simulink model "H8_6GDL_partelinealizada"  (R2022b)
settings: Solver=VariableStepAuto  StartTime=0.0  StopTime=3  RelTol=1e-3
InitFcn:
  | m = 200;
  | g = 9.81;
  | 
  | x_lev12 = 0.443;
  | x_lev34 = 0.542;
  | x_guid12 = 0.4475;
  | x_guid34 = 0.5465;
  | x_lim = 0.0495;
  | 
  | y_lev13 = 0.23686;
  | y_lev24 = 0.23686;
  | y_guid13 = 0.24263;
  | y_guid24 = 0.24263;
  | y_lim = 0.0005;
  | y_brk = 0.21552;
  | 
  | z_lev = 0.08546;
  | z_guid = 0.026;
  | z_lim = 0.1055;
  | z_brk = 0.03941;
  | 
  | kp_lev = 50;
  | ki_lev = 400;
  | kp_guid = 6;
  | ki_guid = 46.5;
  | 
  | Imax_lev = 50;
  | Imin_lev = -50;
  | Imax_guid = 50;
  | Imin_guid = 0;
  | 
  | cg_nom = 0.567;
  | 
  | I = [43.082 0 0; 0 26.887 0; 0 0 29.297]
undefined symbols (not defined in the file or in its folder): ems, hems
libraries: shared6dof x1
settings Model: Creator=aceao  LastModifiedBy=aceao

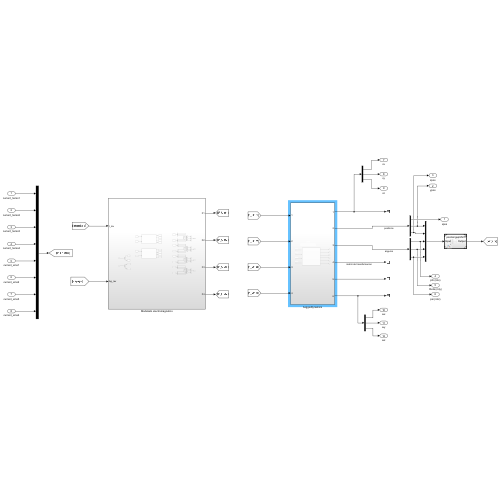
[thumbnail: Simulink's stored preview of the top-level diagram]
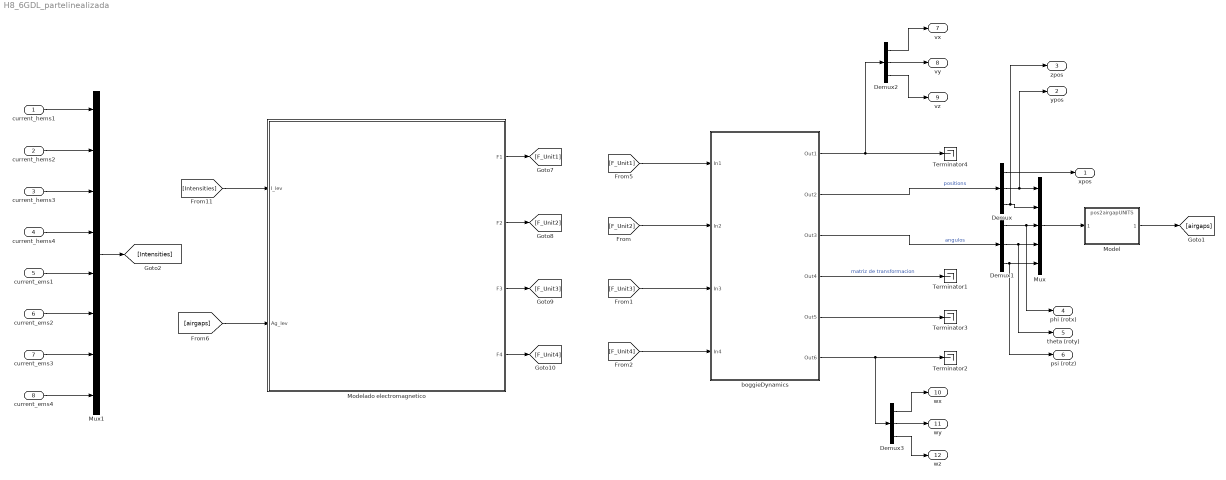
== system H8_6GDL_partelinealizada ==
  current_hems1 : Inport
  current_hems2 : Inport  Port=2
  current_hems3 : Inport  Port=3
  current_hems4 : Inport  Port=4
  current_ems1 : Inport  Port=5
  current_ems2 : Inport  Port=6
  current_ems3 : Inport  Port=7
  current_ems4 : Inport  Port=8
  Demux{,1..3} (4 alike) : Demux  Outputs=3
  Model : ModelReference  ModelNameDialog=pos2airgapUNITS.slx  SimulationMode=Normal  ModelReferenceVersion=1.2
  Modelado electromagnetico : Subsystem
  Mux : Mux  Inputs=5
  Mux1 : Mux  Inputs=8
  Terminator{1..4} (4 alike) : Terminator
  boggieDynamics : Subsystem
  xpos : Outport
  ypos : Outport  Port=2
  zpos : Outport  Port=3
  phi (rotx) : Outport  Port=4
  theta (roty) : Outport  Port=5
  psi (rotz) : Outport  Port=6
  vx : Outport  Port=7
  vy : Outport  Port=8
  vz : Outport  Port=9
  wx : Outport  Port=10
  wy : Outport  Port=11
  wz : Outport  Port=12
  wires:
  Mux1/1 -> [Intensities]
  current_hems2/1 -> Mux1/2
  current_ems3/1 -> Mux1/7
  current_hems4/1 -> Mux1/4
  Modelado electromagnetico/4(F4) -> [F_Unit4]
  current_ems2/1 -> Mux1/6
  current_hems3/1 -> Mux1/3
  current_ems1/1 -> Mux1/5
  current_ems4/1 -> Mux1/8
  current_hems1/1 -> Mux1/1
  Modelado electromagnetico/2(F2) -> [F_Unit2]
  [Intensities] -> Modelado electromagnetico/1(I_lev)
  Modelado electromagnetico/1(F1) -> [F_Unit1]
  Modelado electromagnetico/3(F3) -> [F_Unit3]
  [airgaps] -> Modelado electromagnetico/2(Ag_lev)
  boggieDynamics/2(Out2) -> Demux/1  "positions"
  boggieDynamics/5(Out5) -> Terminator3/1
  Demux1/3 -> psi (rotz)/1, Mux/5
  boggieDynamics/3(Out3) -> Demux1/1  "angulos"
  boggieDynamics/6(Out6) -> Terminator2/1, Demux3/1
  Demux/3 -> zpos/1, Mux/2
  [F_Unit1] -> boggieDynamics/1(In1)
  [F_Unit3] -> boggieDynamics/3(In3)
  Demux/1 -> xpos/1
  boggieDynamics/1(Out1) -> Terminator4/1, Demux2/1
  Mux/1 -> Model/1
  Demux/2 -> Mux/1, ypos/1
  Demux1/1 -> phi (rotx)/1, Mux/3
  [F_Unit2] -> boggieDynamics/2(In2)
  Demux1/2 -> theta (roty)/1, Mux/4
  [F_Unit4] -> boggieDynamics/4(In4)
  boggieDynamics/4(Out4) -> Terminator1/1  "matriz de transformacion"
  Demux2/2 -> vy/1
  Demux2/3 -> vz/1
  Demux3/1 -> wx/1
  Demux3/2 -> wy/1
  Demux3/3 -> wz/1
  Demux2/1 -> vx/1
  Model/1 -> [airgaps]

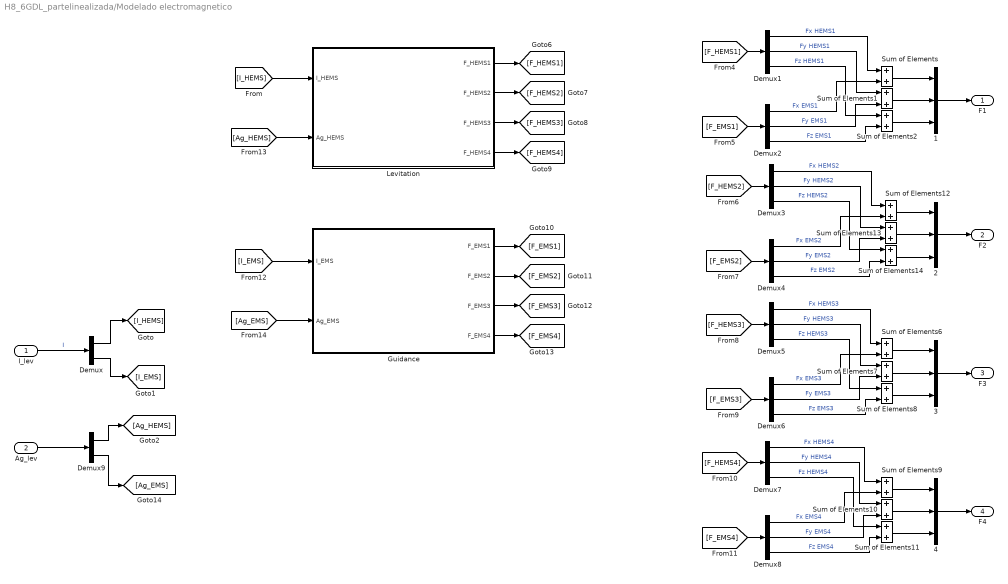
== system H8_6GDL_partelinealizada/Modelado electromagnetico ==
  I_lev : Inport
  Ag_lev : Inport  Port=2
  {1..4} (4 alike) : Mux  Inputs=3
  Demux : Demux  Outputs=2
  Demux{1..8} (8 alike) : Demux  Outputs=3
  Demux9 : Demux  Outputs=2
  Guidance : Subsystem
  Levitation : Subsystem
  Sum of Elements{,1..2,6..14} (12 alike) : Sum
  F1 : Outport
  F2 : Outport  Port=2
  F3 : Outport  Port=3
  F4 : Outport  Port=4
  wires:
  I_lev/1 -> Demux/1  "I"
  Demux/1 -> [I_HEMS]
  Demux/2 -> [I_EMS]
  [I_HEMS] -> Levitation/1(I_HEMS)
  Levitation/1(F_HEMS1) -> [F_HEMS1]
  Levitation/2(F_HEMS2) -> [F_HEMS2]
  Levitation/3(F_HEMS3) -> [F_HEMS3]
  Levitation/4(F_HEMS4) -> [F_HEMS4]
  Sum of Elements/1 -> 1/1
  1/1 -> F1/1
  Sum of Elements1/1 -> 1/2
  Sum of Elements2/1 -> 1/3
  2/1 -> F2/1
  [F_HEMS1] -> Demux1/1
  Demux1/1 -> Sum of Elements/1  "Fx HEMS1"
  Demux1/2 -> Sum of Elements1/1  "Fy HEMS1"
  Demux1/3 -> Sum of Elements2/1  "Fz HEMS1"
  3/1 -> F3/1
  Sum of Elements8/1 -> 3/3
  Sum of Elements6/1 -> 3/1
  Sum of Elements7/1 -> 3/2
  4/1 -> F4/1
  Sum of Elements11/1 -> 4/3
  Sum of Elements9/1 -> 4/1
  Sum of Elements10/1 -> 4/2
  Guidance/2(F_EMS2) -> [F_EMS2]
  Guidance/3(F_EMS3) -> [F_EMS3]
  Guidance/4(F_EMS4) -> [F_EMS4]
  Guidance/1(F_EMS1) -> [F_EMS1]
  Demux2/1 -> Sum of Elements/2  "Fx EMS1"
  [F_EMS1] -> Demux2/1
  Demux2/2 -> Sum of Elements1/2  "Fy EMS1"
  Demux2/3 -> Sum of Elements2/2  "Fz EMS1"
  [F_EMS2] -> Demux4/1
  Demux4/1 -> Sum of Elements12/2  "Fx EMS2"
  Demux4/2 -> Sum of Elements13/2  "Fy EMS2"
  Sum of Elements14/1 -> 2/3
  Demux3/1 -> Sum of Elements12/1  "Fx HEMS2"
  [F_HEMS2] -> Demux3/1
  Demux3/2 -> Sum of Elements13/1  "Fy HEMS2"
  Demux3/3 -> Sum of Elements14/1  "Fz HEMS2"
  Sum of Elements13/1 -> 2/2
  Sum of Elements12/1 -> 2/1
  Demux4/3 -> Sum of Elements14/2  "Fz EMS2"
  Demux5/3 -> Sum of Elements8/1  "Fz HEMS3"
  Demux5/2 -> Sum of Elements7/1  "Fy HEMS3"
  [F_HEMS3] -> Demux5/1
  Demux6/3 -> Sum of Elements8/2  "Fz EMS3"
  [F_EMS3] -> Demux6/1
  Demux6/1 -> Sum of Elements6/2  "Fx EMS3"
  Demux5/1 -> Sum of Elements6/1  "Fx HEMS3"
  Demux6/2 -> Sum of Elements7/2  "Fy EMS3"
  Demux7/3 -> Sum of Elements11/1  "Fz HEMS4"
  Demux8/3 -> Sum of Elements11/2  "Fz EMS4"
  Demux8/2 -> Sum of Elements10/2  "Fy EMS4"
  Demux7/2 -> Sum of Elements10/1  "Fy HEMS4"
  Demux7/1 -> Sum of Elements9/1  "Fx HEMS4"
  Demux8/1 -> Sum of Elements9/2  "Fx EMS4"
  [F_HEMS4] -> Demux7/1
  [F_EMS4] -> Demux8/1
  [I_EMS] -> Guidance/1(I_EMS)
  Ag_lev/1 -> Demux9/1
  Demux9/1 -> [Ag_HEMS]
  Demux9/2 -> [Ag_EMS]
  [Ag_HEMS] -> Levitation/2(Ag_HEMS)
  [Ag_EMS] -> Guidance/2(Ag_EMS)

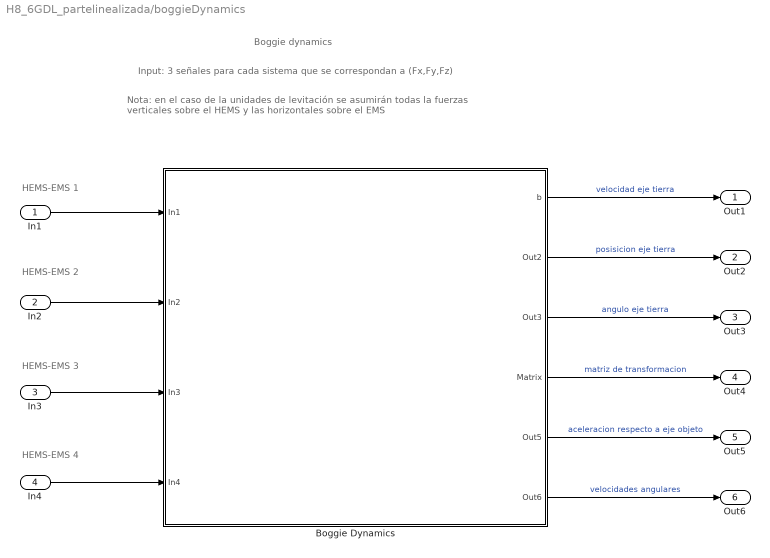
== system H8_6GDL_partelinealizada/boggieDynamics ==
  note: Input: 3 señales para cada sistema que se correspondan a (Fx,Fy,Fz)
  note: HEMS-EMS 3
  note: HEMS-EMS 1
  note: HEMS-EMS 4
  note: HEMS-EMS 2
  note: Boggie dynamics
  note: Nota: en el caso de la unidades de levitación se asumirán todas la fuerzas
      | verticales sobre el HEMS y las horizontales sobre el EMS
  In1 : Inport
  In2 : Inport  Port=2
  In3 : Inport  Port=3
  In4 : Inport  Port=4
  Boggie Dynamics : Subsystem
      mask Display: image('C:\UPV\Hyperloop\Levitacion\ejes.png'); % Use "Edit Image" on toolstrip to change.
  Out1 : Outport
  Out2 : Outport  Port=2
  Out3 : Outport  Port=3
  Out4 : Outport  Port=4
  Out5 : Outport  Port=5
  Out6 : Outport  Port=6
  wires:
  Boggie Dynamics/4(Matrix) -> Out4/1  "matriz de transformacion"
  Boggie Dynamics/6(Out6) -> Out6/1  "velocidades angulares"
  Boggie Dynamics/5(Out5) -> Out5/1  "aceleracion respecto a eje objeto"
  In1/1 -> Boggie Dynamics/1(In1)
  In3/1 -> Boggie Dynamics/3(In3)
  In4/1 -> Boggie Dynamics/4(In4)
  Boggie Dynamics/1(b) -> Out1/1  "velocidad eje tierra"
  In2/1 -> Boggie Dynamics/2(In2)
  Boggie Dynamics/2(Out2) -> Out2/1  "posisicion eje tierra"
  Boggie Dynamics/3(Out3) -> Out3/1  "angulo eje tierra"

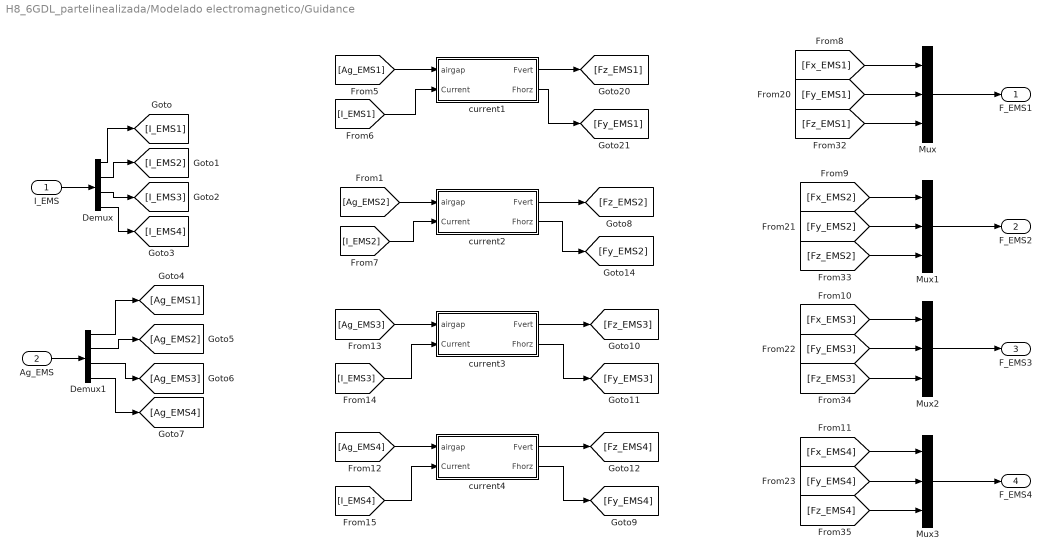
== system H8_6GDL_partelinealizada/Modelado electromagnetico/Guidance ==
  I_EMS : Inport
  Ag_EMS : Inport  Port=2
  Demux : Demux
  Demux1 : Demux
  Mux{,1..3} (4 alike) : Mux  Inputs=3
  current1 : Subsystem
  current2 : Subsystem
  current3 : Subsystem
  current4 : Subsystem
  F_EMS1 : Outport
  F_EMS2 : Outport  Port=2
  F_EMS3 : Outport  Port=3
  F_EMS4 : Outport  Port=4
  wires:
  [Fz_EMS4] -> Mux3/3
  Demux1/4 -> [Ag_EMS4]
  [Fy_EMS1] -> Mux/2
  I_EMS/1 -> Demux/1
  Mux1/1 -> F_EMS2/1
  Demux/2 -> [I_EMS2]
  [Fy_EMS3] -> Mux2/2
  Mux3/1 -> F_EMS4/1
  [Fy_EMS4] -> Mux3/2
  [Fz_EMS1] -> Mux/3
  Mux/1 -> F_EMS1/1
  Mux2/1 -> F_EMS3/1
  [Fx_EMS3] -> Mux2/1
  Demux1/3 -> [Ag_EMS3]
  Ag_EMS/1 -> Demux1/1
  [Fz_EMS3] -> Mux2/3
  Demux/1 -> [I_EMS1]
  [Fz_EMS2] -> Mux1/3
  [Fx_EMS1] -> Mux/1
  Demux1/1 -> [Ag_EMS1]
  Demux/4 -> [I_EMS4]
  [Fx_EMS2] -> Mux1/1
  [Fy_EMS2] -> Mux1/2
  [Fx_EMS4] -> Mux3/1
  Demux/3 -> [I_EMS3]
  Demux1/2 -> [Ag_EMS2]
  current1/1(Fvert) -> [Fz_EMS1]
  current1/2(Fhorz) -> [Fy_EMS1]
  [Ag_EMS1] -> current1/1(airgap)
  [I_EMS1] -> current1/2(Current)
  current2/1(Fvert) -> [Fz_EMS2]
  [Ag_EMS2] -> current2/1(airgap)
  [I_EMS2] -> current2/2(Current)
  current2/2(Fhorz) -> [Fy_EMS2]
  current3/1(Fvert) -> [Fz_EMS3]
  [Ag_EMS3] -> current3/1(airgap)
  current4/1(Fvert) -> [Fz_EMS4]
  [I_EMS3] -> current3/2(Current)
  current4/2(Fhorz) -> [Fy_EMS4]
  current3/2(Fhorz) -> [Fy_EMS3]
  [Ag_EMS4] -> current4/1(airgap)
  [I_EMS4] -> current4/2(Current)

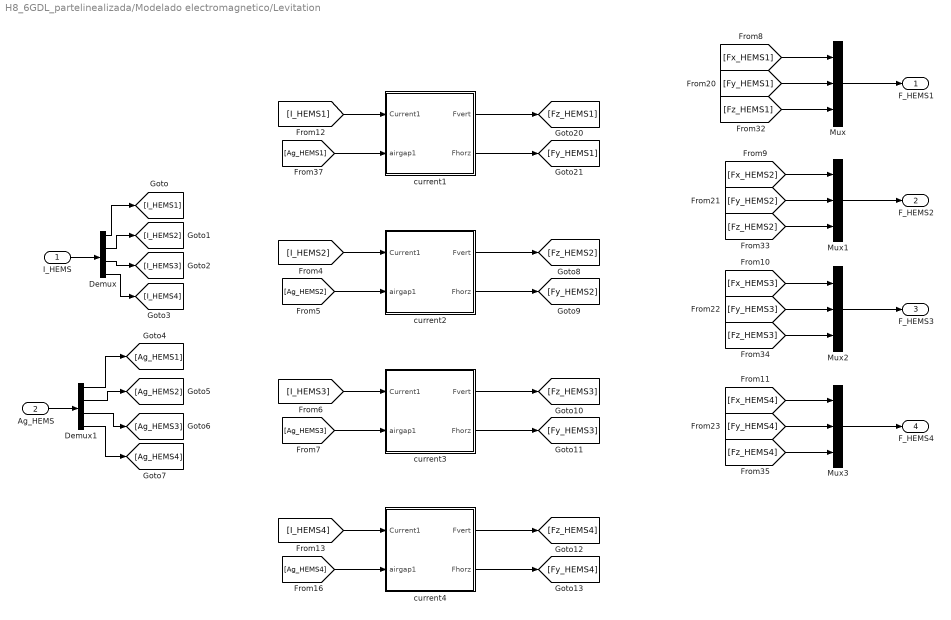
== system H8_6GDL_partelinealizada/Modelado electromagnetico/Levitation ==
  I_HEMS : Inport
  Ag_HEMS : Inport  Port=2
  Demux : Demux
  Demux1 : Demux
  Mux{,1..3} (4 alike) : Mux  Inputs=3
  current1 : Subsystem
  current2 : Subsystem
  current3 : Subsystem
  current4 : Subsystem
  F_HEMS1 : Outport
  F_HEMS2 : Outport  Port=2
  F_HEMS3 : Outport  Port=3
  F_HEMS4 : Outport  Port=4
  wires:
  I_HEMS/1 -> Demux/1
  Mux/1 -> F_HEMS1/1
  Mux1/1 -> F_HEMS2/1
  Mux2/1 -> F_HEMS3/1
  Mux3/1 -> F_HEMS4/1
  Demux/1 -> [I_HEMS1]
  Demux/2 -> [I_HEMS2]
  Demux/3 -> [I_HEMS3]
  Demux/4 -> [I_HEMS4]
  Demux1/2 -> [Ag_HEMS2]
  Demux1/3 -> [Ag_HEMS3]
  Ag_HEMS/1 -> Demux1/1
  Demux1/4 -> [Ag_HEMS4]
  Demux1/1 -> [Ag_HEMS1]
  [Fx_HEMS1] -> Mux/1
  [Fx_HEMS2] -> Mux1/1
  [Fx_HEMS3] -> Mux2/1
  [Fx_HEMS4] -> Mux3/1
  [Fy_HEMS1] -> Mux/2
  [Fy_HEMS2] -> Mux1/2
  [Fy_HEMS3] -> Mux2/2
  [Fy_HEMS4] -> Mux3/2
  [Fz_HEMS1] -> Mux/3
  [Fz_HEMS2] -> Mux1/3
  [Fz_HEMS3] -> Mux2/3
  [Fz_HEMS4] -> Mux3/3
  current1/1(Fvert) -> [Fz_HEMS1]
  current1/2(Fhorz) -> [Fy_HEMS1]
  [I_HEMS1] -> current1/1(Current1)
  [Ag_HEMS1] -> current1/2(airgap1)
  current2/1(Fvert) -> [Fz_HEMS2]
  [Ag_HEMS2] -> current2/2(airgap1)
  current2/2(Fhorz) -> [Fy_HEMS2]
  [I_HEMS2] -> current2/1(Current1)
  current3/1(Fvert) -> [Fz_HEMS3]
  [Ag_HEMS3] -> current3/2(airgap1)
  [I_HEMS4] -> current4/1(Current1)
  [I_HEMS3] -> current3/1(Current1)
  current4/2(Fhorz) -> [Fy_HEMS4]
  current3/2(Fhorz) -> [Fy_HEMS3]
  current4/1(Fvert) -> [Fz_HEMS4]
  [Ag_HEMS4] -> current4/2(airgap1)

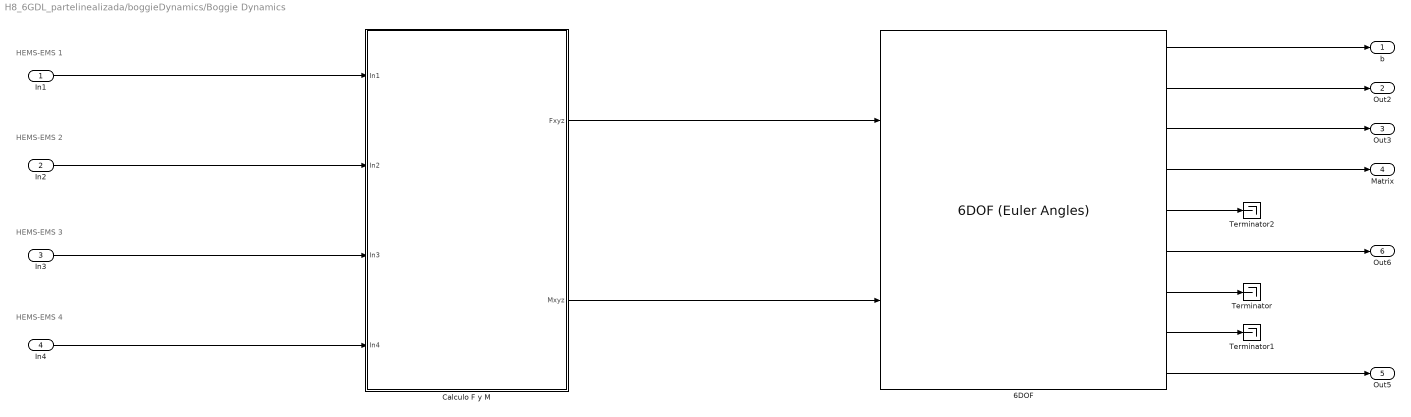
== system H8_6GDL_partelinealizada/boggieDynamics/Boggie Dynamics ==
  note: HEMS-EMS 1
  note: HEMS-EMS 2
  note: HEMS-EMS 3
  note: HEMS-EMS 4
  In1 : Inport
  In2 : Inport  Port=2
  In3 : Inport  Port=3
  In4 : Inport  Port=4
  "6DOF " : shared6dof/6DOF (Euler Angles)  units=Metric (MKS)  mtype=Fixed  rep=Euler Angles  xme_0=[0 0 cg_nom]  Vm_0=[0 0 0]  eul_0=[0 0 0]  pm_0=[0 0 0]  mass_0=m  mass_e=0.5  mass_f=2.0  inertia=I  inertia_e=eye(3)  inertia_f=2*eye(3)  k_quat=1.0  vre_flag=on  abi_flag=on  aMode=0  xme_statename=''  Vm_statename=''  eul_statename=''  quat_statename=''  pm_statename=''  mass_statename=''
  Calculo F y M : Subsystem
  Terminator : Terminator
  Terminator1 : Terminator
  Terminator2 : Terminator
  b : Outport
  Out2 : Outport  Port=2
  Out3 : Outport  Port=3
  Matrix : Outport  Port=4
  Out5 : Outport  Port=5
  Out6 : Outport  Port=6
  wires:
  "6DOF "/1 -> b/1
  "6DOF "/2 -> Out2/1
  "6DOF "/3 -> Out3/1
  In1/1 -> Calculo F y M/1(In1)
  In2/1 -> Calculo F y M/2(In2)
  In3/1 -> Calculo F y M/3(In3)
  In4/1 -> Calculo F y M/4(In4)
  "6DOF "/6 -> Out6/1
  "6DOF "/8 -> Terminator1/1
  "6DOF "/7 -> Terminator/1
  Calculo F y M/1(Fxyz) -> "6DOF "/1
  Calculo F y M/2(Mxyz) -> "6DOF "/2
  "6DOF "/4 -> Matrix/1
  "6DOF "/9 -> Out5/1
  "6DOF "/5 -> Terminator2/1

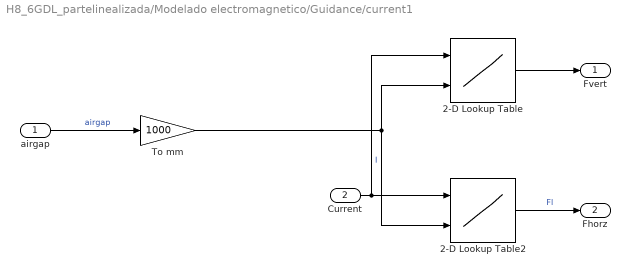
== system H8_6GDL_partelinealizada/Modelado electromagnetico/Guidance/current1 ==
  airgap : Inport
  Current : Inport  Port=2
  2-D Lookup Table : Lookup_n-D  BreakpointsForDimension1=ems.Current  BreakpointsForDimension2=ems.Airgap'  Table=ems.Force_Vertical  InternalRulePriority=Speed  RndMeth=Simplest
      settings: InputPortMap=u0,u1
  2-D Lookup Table2 : Lookup_n-D  BreakpointsForDimension1=ems.Current  BreakpointsForDimension2=ems.Airgap'  Table=ems.Force_Horizontal  InternalRulePriority=Speed  RndMeth=Simplest
      settings: InputPortMap=u0,u1
  To mm : Gain  Gain=1000
  Fvert : Outport
  Fhorz : Outport  Port=2
  wires:
  2-D Lookup Table2/1 -> Fhorz/1  "Fl"
  Current/1 -> 2-D Lookup Table2/1, 2-D Lookup Table/1  "I"
  2-D Lookup Table/1 -> Fvert/1
  airgap/1 -> To mm/1  "airgap"
  To mm/1 -> 2-D Lookup Table/2, 2-D Lookup Table2/2

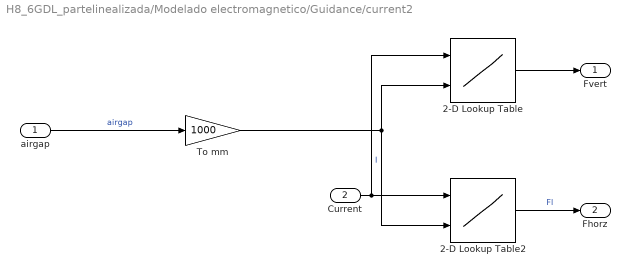
== system H8_6GDL_partelinealizada/Modelado electromagnetico/Guidance/current2 ==
  airgap : Inport
  Current : Inport  Port=2
  2-D Lookup Table : Lookup_n-D  BreakpointsForDimension1=ems.Current  BreakpointsForDimension2=ems.Airgap'  Table=ems.Force_Vertical  InternalRulePriority=Speed  RndMeth=Simplest
      settings: InputPortMap=u0,u1
  2-D Lookup Table2 : Lookup_n-D  BreakpointsForDimension1=ems.Current  BreakpointsForDimension2=ems.Airgap'  Table=ems.Force_Horizontal  InternalRulePriority=Speed  RndMeth=Simplest
      settings: InputPortMap=u0,u1
  To mm : Gain  Gain=1000
  Fvert : Outport
  Fhorz : Outport  Port=2
  wires:
  2-D Lookup Table2/1 -> Fhorz/1  "Fl"
  Current/1 -> 2-D Lookup Table2/1, 2-D Lookup Table/1  "I"
  2-D Lookup Table/1 -> Fvert/1
  airgap/1 -> To mm/1  "airgap"
  To mm/1 -> 2-D Lookup Table2/2, 2-D Lookup Table/2

== system H8_6GDL_partelinealizada/Modelado electromagnetico/Guidance/current3 ==
  airgap : Inport
  Current : Inport  Port=2
  2-D Lookup Table : Lookup_n-D  BreakpointsForDimension1=ems.Current  BreakpointsForDimension2=ems.Airgap'  Table=ems.Force_Vertical  InternalRulePriority=Speed  RndMeth=Simplest
      settings: InputPortMap=u0,u1
  2-D Lookup Table2 : Lookup_n-D  BreakpointsForDimension1=ems.Current  BreakpointsForDimension2=ems.Airgap'  Table=ems.Force_Horizontal  InternalRulePriority=Speed  RndMeth=Simplest
      settings: InputPortMap=u0,u1
  To mm : Gain  Gain=1000
  Fvert : Outport
  Fhorz : Outport  Port=2
  wires:
  2-D Lookup Table2/1 -> Fhorz/1  "Fl"
  Current/1 -> 2-D Lookup Table2/1, 2-D Lookup Table/1  "I"
  2-D Lookup Table/1 -> Fvert/1
  airgap/1 -> To mm/1  "airgap"
  To mm/1 -> 2-D Lookup Table/2, 2-D Lookup Table2/2

== system H8_6GDL_partelinealizada/Modelado electromagnetico/Guidance/current4 ==
  airgap : Inport
  Current : Inport  Port=2
  2-D Lookup Table : Lookup_n-D  BreakpointsForDimension1=ems.Current  BreakpointsForDimension2=ems.Airgap'  Table=ems.Force_Vertical  InternalRulePriority=Speed  RndMeth=Simplest
      settings: InputPortMap=u0,u1
  2-D Lookup Table2 : Lookup_n-D  BreakpointsForDimension1=ems.Current  BreakpointsForDimension2=ems.Airgap'  Table=ems.Force_Horizontal  InternalRulePriority=Speed  RndMeth=Simplest
      settings: InputPortMap=u0,u1
  To mm : Gain  Gain=1000
  Fvert : Outport
  Fhorz : Outport  Port=2
  wires:
  2-D Lookup Table2/1 -> Fhorz/1  "Fl"
  Current/1 -> 2-D Lookup Table2/1, 2-D Lookup Table/1  "I"
  2-D Lookup Table/1 -> Fvert/1
  airgap/1 -> To mm/1  "airgap"
  To mm/1 -> 2-D Lookup Table/2, 2-D Lookup Table2/2

== system H8_6GDL_partelinealizada/Modelado electromagnetico/Levitation/current1 ==
  Current1 : Inport
  airgap1 : Inport  Port=2
  2-D Lookup Table : Lookup_n-D  BreakpointsForDimension1=hems.Airgap'  BreakpointsForDimension2=hems.Current  Table=hems.Force_Vertical  InternalRulePriority=Speed  RndMeth=Simplest
      settings: InputPortMap=u0,u1
  2-D Lookup Table1 : Lookup_n-D  BreakpointsForDimension1=hems.Airgap'  BreakpointsForDimension2=hems.Current  Table=hems.Force_Horizontal  InternalRulePriority=Speed  RndMeth=Simplest
      settings: InputPortMap=u0,u1
  To mm : Gain  Gain=1000
  Fvert : Outport
  Fhorz : Outport  Port=2
  wires:
  2-D Lookup Table1/1 -> Fhorz/1  "Fl"
  2-D Lookup Table/1 -> Fvert/1  "Fl"
  Current1/1 -> 2-D Lookup Table1/2, 2-D Lookup Table/2  "I"
  airgap1/1 -> To mm/1
  To mm/1 -> 2-D Lookup Table1/1, 2-D Lookup Table/1

== system H8_6GDL_partelinealizada/Modelado electromagnetico/Levitation/current2 ==
  Current1 : Inport
  airgap1 : Inport  Port=2
  2-D Lookup Table : Lookup_n-D  BreakpointsForDimension1=hems.Airgap'  BreakpointsForDimension2=hems.Current  Table=hems.Force_Vertical  InternalRulePriority=Speed  RndMeth=Simplest
      settings: InputPortMap=u0,u1
  2-D Lookup Table1 : Lookup_n-D  BreakpointsForDimension1=hems.Airgap'  BreakpointsForDimension2=hems.Current  Table=hems.Force_Horizontal  InternalRulePriority=Speed  RndMeth=Simplest
      settings: InputPortMap=u0,u1
  To mm : Gain  Gain=1000
  Fvert : Outport
  Fhorz : Outport  Port=2
  wires:
  2-D Lookup Table1/1 -> Fhorz/1  "Fl"
  2-D Lookup Table/1 -> Fvert/1  "Fl"
  Current1/1 -> 2-D Lookup Table1/2, 2-D Lookup Table/2  "I"
  airgap1/1 -> To mm/1
  To mm/1 -> 2-D Lookup Table1/1, 2-D Lookup Table/1

== system H8_6GDL_partelinealizada/Modelado electromagnetico/Levitation/current3 ==
  Current1 : Inport
  airgap1 : Inport  Port=2
  2-D Lookup Table : Lookup_n-D  BreakpointsForDimension1=hems.Airgap'  BreakpointsForDimension2=hems.Current  Table=hems.Force_Vertical  InternalRulePriority=Speed  RndMeth=Simplest
      settings: InputPortMap=u0,u1
  2-D Lookup Table1 : Lookup_n-D  BreakpointsForDimension1=hems.Airgap'  BreakpointsForDimension2=hems.Current  Table=hems.Force_Horizontal  InternalRulePriority=Speed  RndMeth=Simplest
      settings: InputPortMap=u0,u1
  To mm : Gain  Gain=1000
  Fvert : Outport
  Fhorz : Outport  Port=2
  wires:
  2-D Lookup Table1/1 -> Fhorz/1  "Fl"
  2-D Lookup Table/1 -> Fvert/1  "Fl"
  Current1/1 -> 2-D Lookup Table1/2, 2-D Lookup Table/2  "I"
  airgap1/1 -> To mm/1
  To mm/1 -> 2-D Lookup Table1/1, 2-D Lookup Table/1

== system H8_6GDL_partelinealizada/Modelado electromagnetico/Levitation/current4 ==
  Current1 : Inport
  airgap1 : Inport  Port=2
  2-D Lookup Table : Lookup_n-D  BreakpointsForDimension1=hems.Airgap'  BreakpointsForDimension2=hems.Current  Table=hems.Force_Vertical  InternalRulePriority=Speed  RndMeth=Simplest
      settings: InputPortMap=u0,u1
  2-D Lookup Table1 : Lookup_n-D  BreakpointsForDimension1=hems.Airgap'  BreakpointsForDimension2=hems.Current  Table=hems.Force_Horizontal  InternalRulePriority=Speed  RndMeth=Simplest
      settings: InputPortMap=u0,u1
  To mm : Gain  Gain=1000
  Fvert : Outport
  Fhorz : Outport  Port=2
  wires:
  2-D Lookup Table1/1 -> Fhorz/1  "Fl"
  2-D Lookup Table/1 -> Fvert/1  "Fl"
  Current1/1 -> 2-D Lookup Table1/2, 2-D Lookup Table/2  "I"
  airgap1/1 -> To mm/1
  To mm/1 -> 2-D Lookup Table1/1, 2-D Lookup Table/1

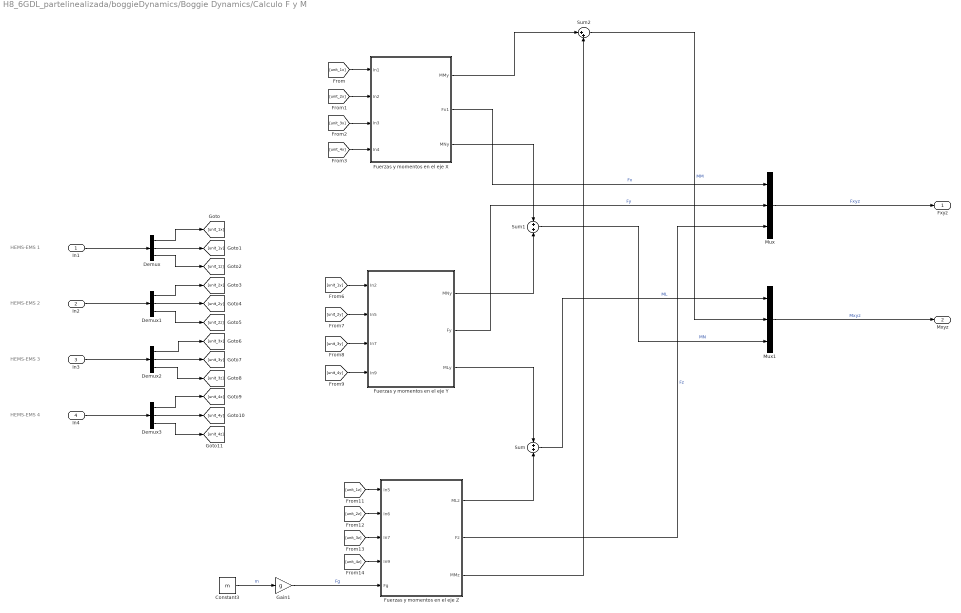
== system H8_6GDL_partelinealizada/boggieDynamics/Boggie Dynamics/Calculo F y M ==
  note: HEMS-EMS 3
  note: HEMS-EMS 1
  note: HEMS-EMS 4
  note: HEMS-EMS 2
  In1 : Inport
  In2 : Inport  Port=2
  In3 : Inport  Port=3
  In4 : Inport  Port=4
  Constant3 : Constant  Value=m
  Demux{,1..3} (4 alike) : Demux  Outputs=3
  Fuerzas y momentos en el eje X : Subsystem
  Fuerzas y momentos en el eje Y : Subsystem
  Fuerzas y momentos en el eje Z : Subsystem
  Gain1 : Gain  Gain=g
  Mux : Mux  Inputs=3
  Mux1 : Mux  Inputs=3
  Sum : Sum
  Sum1 : Sum
  Sum2 : Sum  Inputs=|++
  Fxyz : Outport
  Mxyz : Outport  Port=2
  wires:
  In3/1 -> Demux2/1
  Constant3/1 -> Gain1/1  "m"
  Sum2/1 -> Mux1/2  "MM"
  Mux/1 -> Fxyz/1  "Fxyz"
  In4/1 -> Demux3/1
  Mux1/1 -> Mxyz/1  "Mxyz"
  Sum1/1 -> Mux1/3  "MN"
  Sum/1 -> Mux1/1  "ML"
  In2/1 -> Demux1/1
  In1/1 -> Demux/1
  Fuerzas y momentos en el eje X/1(MMy) -> Sum2/1
  Fuerzas y momentos en el eje X/2(Fx1) -> Mux/1  "Fx"
  Fuerzas y momentos en el eje X/3(MNy) -> Sum1/1
  Fuerzas y momentos en el eje Y/2(Fy) -> Mux/2  "Fy"
  Fuerzas y momentos en el eje Y/1(MNy) -> Sum1/2
  Fuerzas y momentos en el eje Y/3(MLy) -> Sum/1
  Gain1/1 -> Fuerzas y momentos en el eje Z/5(Fg)  "Fg"
  Fuerzas y momentos en el eje Z/2(Fz) -> Mux/3  "Fz"
  Fuerzas y momentos en el eje Z/1(MLz) -> Sum/2
  Demux3/1 -> [unit_4x]
  Demux3/2 -> [unit_4y]
  Demux3/3 -> [unit_4z]
  Demux2/1 -> [unit_3x]
  Demux2/2 -> [unit_3y]
  Demux2/3 -> [unit_3z]
  Demux1/1 -> [unit_2x]
  Demux1/2 -> [unit_2y]
  Demux1/3 -> [unit_2z]
  Demux/1 -> [unit_1x]
  Demux/2 -> [unit_1y]
  Demux/3 -> [unit_1z]
  [unit_1x] -> Fuerzas y momentos en el eje X/1(In1)
  [unit_2x] -> Fuerzas y momentos en el eje X/2(In2)
  [unit_3x] -> Fuerzas y momentos en el eje X/3(In3)
  [unit_4x] -> Fuerzas y momentos en el eje X/4(In4)
  [unit_4y] -> Fuerzas y momentos en el eje Y/4(In9)
  [unit_1y] -> Fuerzas y momentos en el eje Y/1(In2)
  [unit_2y] -> Fuerzas y momentos en el eje Y/2(In5)
  [unit_3y] -> Fuerzas y momentos en el eje Y/3(In7)
  [unit_1z] -> Fuerzas y momentos en el eje Z/1(In5)
  [unit_3z] -> Fuerzas y momentos en el eje Z/3(In7)
  [unit_2z] -> Fuerzas y momentos en el eje Z/2(In6)
  [unit_4z] -> Fuerzas y momentos en el eje Z/4(In9)
  Fuerzas y momentos en el eje Z/3(MMz) -> Sum2/2

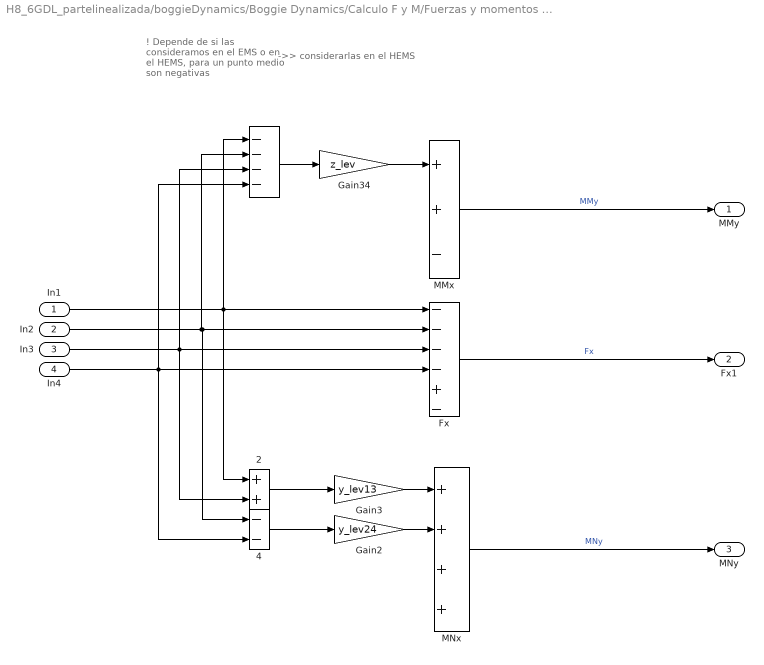
== system H8_6GDL_partelinealizada/boggieDynamics/Boggie Dynamics/Calculo F y M/Fuerzas y momentos en el eje X ==
  note: ! Depende de si las consideramos en el EMS o en el HEMS,
      | para un punto medio son negativas
  note: ->> considerarlas en el HEMS
  In1 : Inport
  In2 : Inport  Port=2
  In3 : Inport  Port=3
  In4 : Inport  Port=4
  " " : Sum  Inputs=----
  " 2" : Sum
  " 4" : Sum  Inputs=--
  Fx : Sum  Inputs=----+-
  Gain2 : Gain  Gain=y_lev24
  Gain3 : Gain  Gain=y_lev13
  Gain34 : Gain  Gain=z_lev
  MMx : Sum  Inputs=++-
  MNx : Sum  Inputs=++++
  MMy : Outport
  Fx1 : Outport  Port=2
  MNy : Outport  Port=3
  wires:
  In1/1 -> " 2"/1, " "/1, Fx/1
  In2/1 -> " "/2, " 4"/1, Fx/2
  Fx/1 -> Fx1/1  "Fx"
  MMx/1 -> MMy/1  "MMy"
  In4/1 -> " 4"/2, " "/4, Fx/4
  In3/1 -> " "/3, " 2"/2, Fx/3
  Gain34/1 -> MMx/1
  MNx/1 -> MNy/1  "MNy"
  " "/1 -> Gain34/1
  " 4"/1 -> Gain2/1
  " 2"/1 -> Gain3/1
  Gain3/1 -> MNx/1
  Gain2/1 -> MNx/2

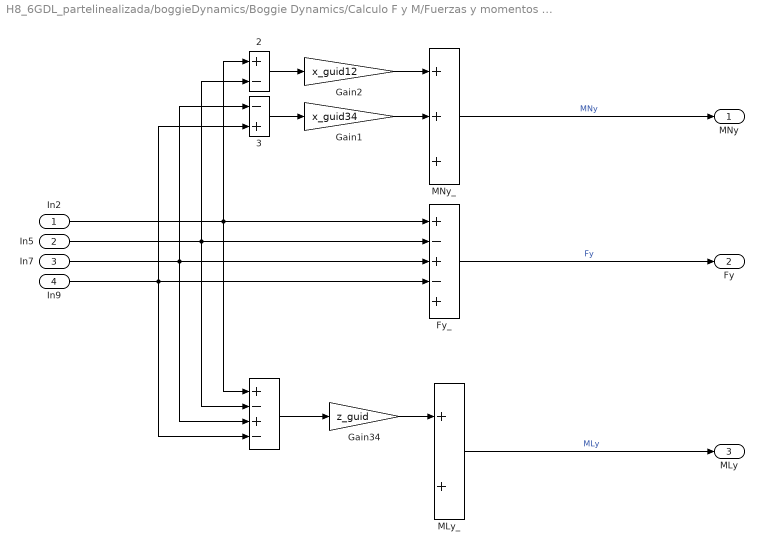
== system H8_6GDL_partelinealizada/boggieDynamics/Boggie Dynamics/Calculo F y M/Fuerzas y momentos en el eje Y ==
  In2 : Inport
  In5 : Inport  Port=2
  In7 : Inport  Port=3
  In9 : Inport  Port=4
  " " : Sum  Inputs=+-+-
  " 2" : Sum  Inputs=+-
  " 3" : Sum  Inputs=-+
  Fy_ : Sum  Inputs=+-+-+
  Gain1 : Gain  Gain=x_guid34
  Gain2 : Gain  Gain=x_guid12
  Gain34 : Gain  Gain=z_guid
  MLy_ : Sum
  MNy_ : Sum  Inputs=+++
  MNy : Outport
  Fy : Outport  Port=2
  MLy : Outport  Port=3
  wires:
  Fy_/1 -> Fy/1  "Fy"
  MLy_/1 -> MLy/1  "MLy"
  In7/1 -> Fy_/3, " "/3, " 3"/1
  In9/1 -> " "/4, " 3"/2, Fy_/4
  In2/1 -> " "/1, " 2"/1, Fy_/1
  In5/1 -> " "/2, Fy_/2, " 2"/2
  MNy_/1 -> MNy/1  "MNy"
  " 3"/1 -> Gain1/1
  " 2"/1 -> Gain2/1
  Gain1/1 -> MNy_/2
  Gain2/1 -> MNy_/1
  " "/1 -> Gain34/1
  Gain34/1 -> MLy_/1

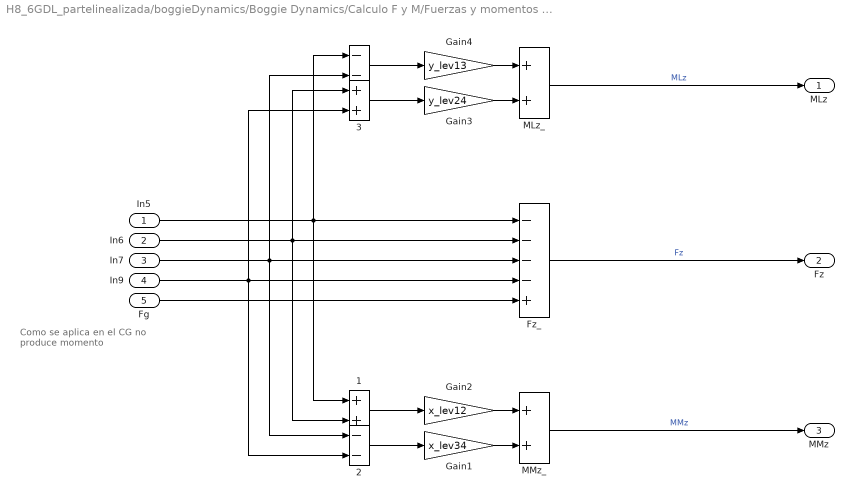
== system H8_6GDL_partelinealizada/boggieDynamics/Boggie Dynamics/Calculo F y M/Fuerzas y momentos en el eje Z ==
  note: Como se aplica en el CG
      |  no produce momento
  In5 : Inport
  In6 : Inport  Port=2
  In7 : Inport  Port=3
  In9 : Inport  Port=4
  Fg : Inport  Port=5
  " " : Sum  Inputs=--
  " 1" : Sum
  " 2" : Sum  Inputs=--
  " 3" : Sum
  " MLz_" : Sum
  " MMz_" : Sum
  Fz_ : Sum  Inputs=----+
  Gain1 : Gain  Gain=x_lev34
  Gain2 : Gain  Gain=x_lev12
  Gain3 : Gain  Gain=y_lev24
  Gain4 : Gain  Gain=y_lev13
  MLz : Outport
  Fz : Outport  Port=2
  MMz : Outport  Port=3
  wires:
  In6/1 -> " 1"/2, Fz_/2, " 3"/1
  " MLz_"/1 -> MLz/1  "MLz"
  Fg/1 -> Fz_/5
  In9/1 -> Fz_/4, " 2"/2, " 3"/2
  In5/1 -> " 1"/1, " "/1, Fz_/1
  In7/1 -> " 2"/1, Fz_/3, " "/2
  Fz_/1 -> Fz/1  "Fz"
  " MMz_"/1 -> MMz/1  "MMz"
  " 3"/1 -> Gain3/1
  " "/1 -> Gain4/1
  Gain4/1 -> " MLz_"/1
  Gain3/1 -> " MLz_"/2
  Gain2/1 -> " MMz_"/1
  " 2"/1 -> Gain1/1
  Gain1/1 -> " MMz_"/2
  " 1"/1 -> Gain2/1
